simulink subsystem "NL_subbloc"  (R2020a)
settings: Solver=VariableStepAuto  StartTime=0.0  StopTime=10.0  RelTol=1e-3
values from neighbouring files (symbols this model uses):
  a = 1    [Adap.m]    (also in Adaptive_control_Non_linear.m = 2; HOSM.m; projet_AAV.m; sys.m)
  b = 2    [Adaptive_Control_Linear.m]    (also in Adaptive_control_Non_linear.m; HOSM.m = 1; feedback-integrator.m = 3; mini_projet.m = 3)
libraries: simulink x1
settings Model: Creator=lenovo  LastModifiedBy=lenovo

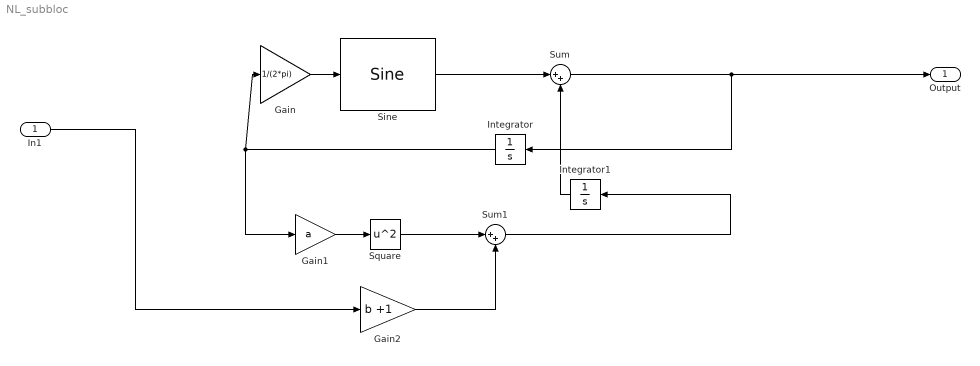
== system NL_subbloc ==
  In1 : Inport
  Gain : Gain  Gain=1/(2*pi)
  Gain1 : Gain  Gain=a
  Gain2 : Gain  Gain=b +1
  Integrator : Integrator
  Integrator1 : Integrator
  Sine : simulink/Lookup Tables/Sine  Formula=sin(2*pi*u)  NumDataPoints=(2^5)+1  OutputWordLength=16  InternalRulePriority=Speed
  Square : Math  Operator=square  SaturateOnIntegerOverflow=on
  Sum : Sum  Inputs=|++
  Sum1 : Sum  Inputs=|++
  Output : Outport
  wires:
  Gain/1 -> Sine/1
  Sine/1 -> Sum/1
  Sum/1 -> Output/1, Integrator/1
  Integrator/1 -> Gain1/1, Gain/1
  Gain1/1 -> Square/1
  Square/1 -> Sum1/1
  Gain2/1 -> Sum1/2
  In1/1 -> Gain2/1
  Sum1/1 -> Integrator1/1
  Integrator1/1 -> Sum/2
